simulink model "ADRC_Control"  (R2022a)
settings: Solver=ode45  StartTime=0.0  StopTime=900  RelTol=1e-3
undefined symbols (not defined in the file or in its folder): path
settings Model: Creator=45489  LastModifiedBy=45489
settings SolverCC: AlgebraicLoopSolver=TrustRegion
settings DebuggingCC: UnconnectedInputMsg=warning  UnconnectedOutputMsg=warning  UnconnectedLineMsg=warning  SFMachineParentedDataDiag=warning

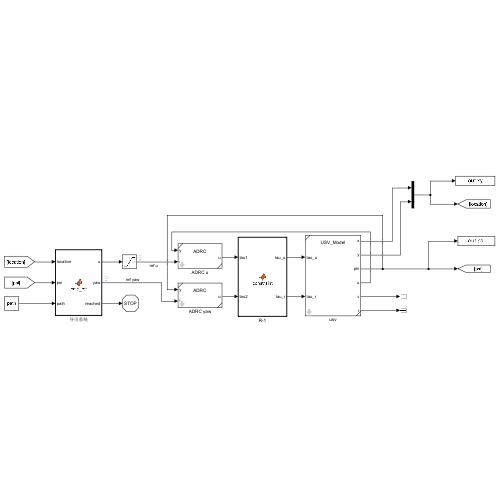
[thumbnail: Simulink's stored preview of the top-level diagram]
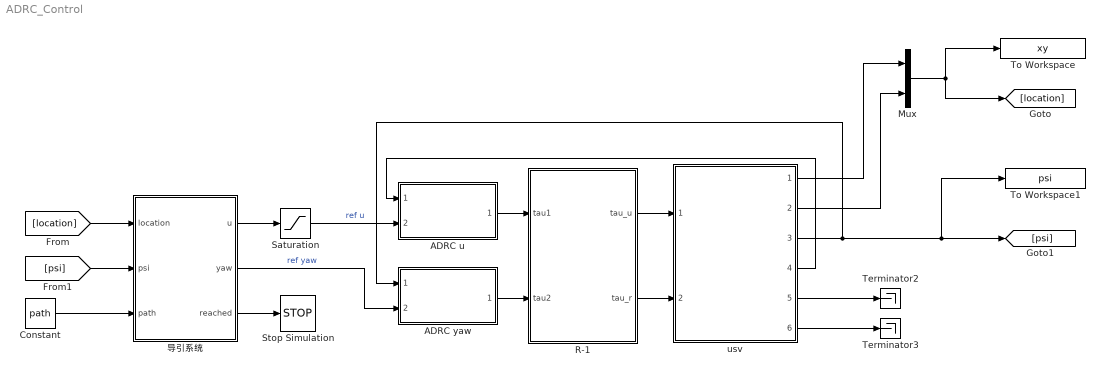
== system ADRC_Control ==
  ADRC u : Subsystem  ReferencedSubsystem=ADRC  para=para_u
  ADRC yaw : Subsystem  ReferencedSubsystem=ADRC  para=para_yaw
  Constant : Constant  Value=path
  Mux : Mux  Inputs=2
  R-1 : MATLAB Function  TreatAsAtomicUnit=on
  Saturation : Saturate  UpperLimit=10  LowerLimit=0.1
  Stop Simulation : Stop
  Terminator2 : Terminator
  Terminator3 : Terminator
  To Workspace : ToWorkspace  VariableName=xy  SaveFormat=Timeseries  SampleTime=-1
  To Workspace1 : ToWorkspace  VariableName=psi  SaveFormat=Timeseries  SampleTime=-1
  usv : Subsystem  ReferencedSubsystem=USV_Model  x=init_x  y=init_y  psi=init_psi
  导引系统 : MATLAB Function  TreatAsAtomicUnit=on
  wires:
  usv/3 -> To Workspace1/1, [psi], ADRC yaw/1
  usv/4 -> ADRC u/1
  usv/5 -> Terminator2/1
  usv/6 -> Terminator3/1
  ADRC u/1 -> R-1/1(tau1)
  ADRC yaw/1 -> R-1/2(tau2)
  R-1/2(tau_r) -> usv/2
  R-1/1(tau_u) -> usv/1
  导引系统/2(yaw) -> ADRC yaw/2  "ref yaw"
  usv/1 -> Mux/1
  usv/2 -> Mux/2
  [location] -> 导引系统/1(location)
  Constant/1 -> 导引系统/3(path)
  [psi] -> 导引系统/2(psi)
  导引系统/1(u) -> Saturation/1
  Saturation/1 -> ADRC u/2  "ref u"
  导引系统/3(reached) -> Stop Simulation/1
  Mux/1 -> [location], To Workspace/1

== matlab function ADRC_Control/导引系统 ==
  settings: updateMethod=DISCRETE
  data: u output size=1; location input size=[2 1]; psi input size=1; yaw output size=1; path input; reached output
function [u, yaw, reached] = calc_ref(location,psi, path)
% u: 期望速度
% yaw: 期望船角度
% reached: 是否到达终点
u=0.1;
yaw=0;
reached=false;

%% 确定目标点
% the closest point which has't been accessed 
persistent k;
if isempty(k)
    k=1;
end

while k<length(path)
    target=path(k,:);
    d=target-location'; % 期望更新矢量
    if sum(d.^2)<25 && k<length(path) % 5m 之内视为已观测, 移到下一个点
       k=k+1;
    else
        break;
    end
end

d=path(k,:)-location'; % 期望更新矢量
if sum(d.^2)<4 % 船距离终点2米, 视为到达终点, 停下来
    u=0;
    yaw=0;
    reached=true;
    return
end

%% 计算期望值
% calculate yaw
yaw=calc_yaw(d);
while abs(yaw-psi)>pi
    if yaw-psi>pi
        yaw=yaw-2*pi;
    elseif yaw-psi<-pi
        yaw=yaw+2*pi;
    end
end

% 如果发现目标点在船的后面(有跟踪失败的风险),则策略切换到选择最近点作为目标点
if abs(yaw-psi)>0.5*pi
    subpath=path(k:end,:);
    dir=subpath-location';
    distance=sum(dir.^2,2); % x^2+y^2
    min_index = find(distance==min(distance));
    k=k + min_index(1)-1; % 找到第一个距离最近的索引, 并转化成相对path的索引
    % 切换 k, 下次更新
end

% calculate u
u=log10(sqrt(sum(d.^2,"all"))+1)*(1+cos(yaw-psi))*0.5; % 考虑到距离, 转角确定速度

function yaw=calc_yaw(d)
    yaw=0;
    if d(1)>0
        yaw=atan(d(2)/d(1));
    elseif d(1)<=0 && d(2) >0
        yaw=pi+atan(d(2)/d(1));
    elseif d(1)<=0 && d(2)<=0
        yaw=-pi+atan(d(2)/d(1));
    end

== matlab function ADRC_Control/R-1 ==
  data: tau1 input; tau_u output; tau2 input; tau_r output
function [tau_u,tau_r] = constraint(tau1,tau2)
B=[1 1; 1 -1];
F=B\[tau1; tau2]; %由总推力和转矩反解左右推力
% 设定 F 最大值 50, 最小值 0.
F(F>50)=50;
F(F<0)=0;
% 恢复为总推力和转矩
tau=B*F;
tau_u=tau(1);tau_r=tau(2);
